simulink model "PID Controller"  (R2021a)
settings: Solver=VariableStepAuto  StartTime=0.0  StopTime=20  MaxStep=.01  RelTol=1e-3
settings Model: Creator=haden  LastModifiedBy=haden

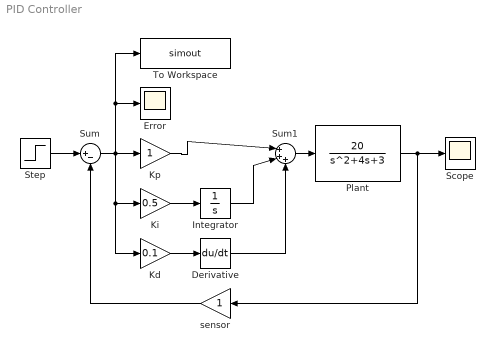
== system PID Controller ==
  Derivative : Derivative
  Error : Scope
  Integrator : Integrator
  Kd : Gain  Gain=0.1
  Ki : Gain  Gain=0.5
  Kp : Gain
  Plant : TransferFcn  Numerator=[20]  Denominator=[1 4 3]
  Scope : Scope
  Step : Step  SampleTime=0
  Sum : Sum  Inputs=|+-
  Sum1 : Sum  Inputs=|+++
  To Workspace : ToWorkspace  VariableName=simout  SaveFormat=Structure With Time  SampleTime=-1
  sensor : Gain
  wires:
  Plant/1 -> sensor/1, Scope/1
  Step/1 -> Sum/1
  sensor/1 -> Sum/2
  Kd/1 -> Derivative/1
  Sum1/1 -> Plant/1
  Ki/1 -> Integrator/1
  Kp/1 -> Sum1/1
  Integrator/1 -> Sum1/2
  Derivative/1 -> Sum1/3
  Sum/1 -> To Workspace/1, Error/1, Ki/1, Kd/1, Kp/1
